simulink model "segway1"  (R2013a)
settings: Solver=ode45  StartTime=0.0  StopTime=10.0  RelTol=1e-3
values from neighbouring files (symbols this model uses):
  m = 0.05    [variables_set.m]
undefined symbols (not defined in the file or in its folder): Assem1, mass, platform, RootGround, RootPart, wheel
libraries: mblibv1 x13
settings Model: Creator=Raja  LastModifiedBy=Raja
settings SimMechanicsCC: VisOnUpdateDiagram=on  VisDuringSimulation=on

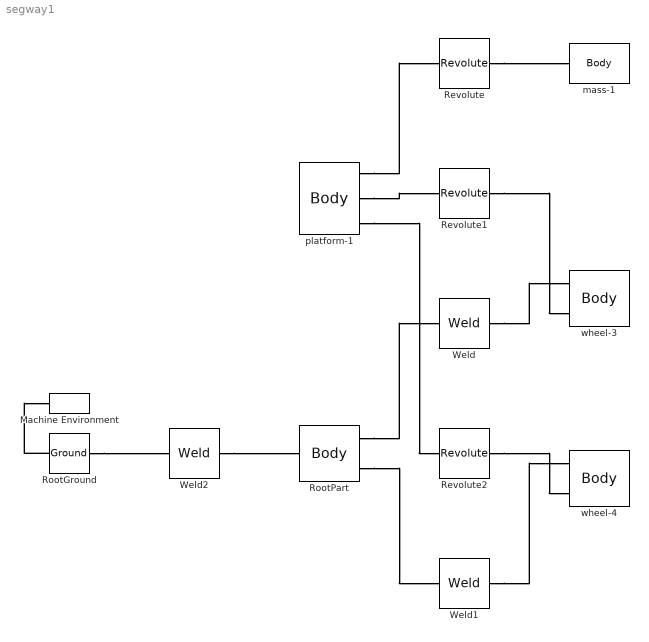
== system segway1 ==
  Machine Environment : mblibv1/Bodies/Machine Environment  PortType=env  PhysicalDomain=Mechanical  DialogTemplateClass=MECH.MachineEnvironment  SyncWhenCopied=off  Gravity=[0 -9.81 0]  GravityUnits=m/s^2  GravityAsSignal=off  Dimensionality=Auto-detect  AnalysisType=Forward dynamics  LinearAssemblyTolerance=1e-3  LinearAssemblyToleranceUnits=m  AngularAssemblyTolerance=1e-3  AngularAssemblyToleranceUnits=rad  ConstraintSolverType=Stabilizing  ConstraintRelTolerance=1e-4  ConstraintAbsTolerance=1e-4  UseRobustSingularityHandling=off  RedundancyAnalysisToleranceType=Automatically select tolerance  RedundancyAnalysisTolerance=1e-14  StatePerturbationType=Fixed  PerturbationSize=1e-5  VisualizeMachine=on  BodyVisualizationType=Use model default body geometries  BodyColorSelMode=Use model default  DefaultBodyColor=[1 0 0]
  Revolute : mblibv1/Joints/Revolute  LConnTagsString=__newl0  RConnTagsString=__newr0  UpdateFromCAD=on  PMImportedID=mass-1:-:platform-1  NumSAPorts=0  CutJoint=off  MarkAsCut=off  Primitives=prismatic  PrimitiveProps=R1$WORLD$[0,0.999884,-0.0152006]$revolute  DialogClass=JointBlock  R1Axis=[0,0.999884,-0.0152006]
  Revolute1 : mblibv1/Joints/Revolute  LConnTagsString=__newl0  RConnTagsString=__newr0  UpdateFromCAD=on  PMImportedID=platform-1:-:wheel-3  NumSAPorts=0  CutJoint=off  MarkAsCut=off  Primitives=prismatic  PrimitiveProps=R1$WORLD$[1,0,0]$revolute  DialogClass=JointBlock  R1Axis=[1,0,0]
  Revolute2 : mblibv1/Joints/Revolute  LConnTagsString=__newl0  RConnTagsString=__newr0  UpdateFromCAD=on  PMImportedID=platform-1:-:wheel-4  NumSAPorts=0  CutJoint=off  MarkAsCut=off  Primitives=prismatic  PrimitiveProps=R1$WORLD$[-1,0,0]$revolute  DialogClass=JointBlock  R1Axis=[-1,0,0]
  RootGround : mblibv1/Bodies/Ground  UpdateFromCAD=on  PMImportedID=RootGround  LeftPortType=env  RightPortType=workingframe  PhysicalDomain=Mechanical  DialogClass=GroundBlock  CoordPosition=[0,0.276214,-0.00378102]  CoordPositionUnits=m  StateVectorMgrId=-1  MachineId=[0 0]  ShowEnvPort=on
  RootPart : mblibv1/Bodies/Body  LConnTagsString=CS4  RConnTagsString=CS2|CS3  UpdateFromCAD=on  PMImportedID=Assem1/RootPart  DialogClass=MechanicalBodyBlock  Mass=0  MassUnits=kg  InertiaUnits=kg*m^2  Inertia=[0,0,0;0,0,0;0,0,0]  Shape=Cylinder  ShapeDims=[1 1]  ShapeUnits=m  ShapeUse=false  Density=1  DensityUnits=kg/m^3  DensityUse=false  GraphicsMode=MACHINE_DEFAULT  BodyColorSelMode=MACHINE_DEFAULT  BodyColor=[1;0;0]  AttachedToCS=CS1  CG=Right$CG$[0 0.276214 -0.00378102]$WORLD$WORLD$m$[1 0 0;0 1 0;0 0 1]$3x3 Transform$rad$WORLD$false$Assem1/RootPart::CG(AUTOGEN)  WorkingFrames=Right$CS1$[0 0 0]$WORLD$WORLD$m$[1 0 0;0 1 0;0 0 1]$3x3 Transform$rad$WORLD$false$Assem1/RootPart::CS1(AUTOGEN)#Right$CS2$[-0.15 0.0275 0]$WORLD$WORLD$m$[1 0 0;0 1 0;0 0 1]$3x3 Transform$rad$WORLD$true$Assem1/RootPart:-:wheel-3::Assem1/RootPart(AUTOGEN)#Right$CS3$[0.15 0.0275 0]$WORLD$WORLD$m$[1 0 0;0 1 0;0 0 1]$3x3 Transform$rad$WORLD$true$Assem1/RootPart:-:wheel-4::Assem1/RootPart(AUTOGEN)#Left$CS4$[0 0.276214 -0.00378102]$WORLD$WORLD$m$[1 0 0;0 1 0;0 0 1]$3x3 Transform$rad$WORLD$true$Assem1/RootPart:-:RootGround::Assem1/RootPart(AUTOGEN)  CGPos=[0 0.276214 -0.00378102]  CGRot=[1 0 0;0 1 0;0 0 1]  CS0Pos=[]  CS0Rot=[]  CS1Pos=[0 0 0]  CS1Rot=[1 0 0;0 1 0;0 0 1]  CS2Pos=[-0.15 0.0275 0]  CS2Rot=[1 0 0;0 1 0;0 0 1]  CS3Pos=[0.15 0.0275 0]  CS3Rot=[1 0 0;0 1 0;0 0 1]  CS4Pos=[0 0.276214 -0.00378102]  CS4Rot=[1 0 0;0 1 0;0 0 1]  CS5Pos=[]  CS5Rot=[]  CS6Pos=[]  CS6Rot=[]  CS7Pos=[]  CS7Rot=[]  CS8Pos=[]  CS8Rot=[]  CS9Pos=[]  CS9Rot=[]  CS10Pos=[]  CS10Rot=[]  CS11Pos=[]  CS11Rot=[]  CS12Pos=[]  CS12Rot=[]  CS13Pos=[]  CS13Rot=[]  CS14Pos=[]  CS14Rot=[]  CS15Pos=[]  CS15Rot=[]  CS16Pos=[]  CS16Rot=[]  CS17Pos=[]  CS17Rot=[]  CS18Pos=[]  CS18Rot=[]  CS19Pos=[]  CS19Rot=[]  CS20Pos=[]  CS20Rot=[]
  Weld : mblibv1/Joints/Weld  LConnTagsString=__newl0  RConnTagsString=__newr0  UpdateFromCAD=on  PMImportedID=Assem1/RootPart:-:wheel-3  NumSAPorts=0  CutJoint=off  MarkAsCut=off  Primitives=weld  PrimitiveProps=W$WORLD$[0.57735,0.57735,0.57735]$weld  DialogClass=JointBlock  WAxis=[0.57735,0.57735,0.57735]
  Weld1 : mblibv1/Joints/Weld  LConnTagsString=__newl0  RConnTagsString=__newr0  UpdateFromCAD=on  PMImportedID=Assem1/RootPart:-:wheel-4  NumSAPorts=0  CutJoint=off  MarkAsCut=off  Primitives=weld  PrimitiveProps=W$WORLD$[0.57735,0.57735,0.57735]$weld  DialogClass=JointBlock  WAxis=[0.57735,0.57735,0.57735]
  Weld2 : mblibv1/Joints/Weld  LConnTagsString=__newl0  RConnTagsString=__newr0  UpdateFromCAD=on  PMImportedID=Assem1/RootPart:-:RootGround  NumSAPorts=0  CutJoint=off  MarkAsCut=off  Primitives=weld  PrimitiveProps=W$WORLD$[0.57735,0.57735,0.57735]$weld  DialogClass=JointBlock  WAxis=[0.57735,0.57735,0.57735]
  mass-1 : mblibv1/Bodies/Body  LConnTagsString=CS2  UpdateFromCAD=on  PMImportedID=mass-1  DialogClass=MechanicalBodyBlock  Mass=0.994043  MassUnits=kg  InertiaUnits=kg*m^2  Inertia=[0.000433605,0,0;0,0.000718103,0;0,0,0.000433605]  Shape=Cylinder  ShapeDims=[1 1]  ShapeUnits=m  ShapeUse=false  Density=1  DensityUnits=kg/m^3  DensityUse=false  GraphicsMode=GFXFILE  GraphicsFileName=Assem1 - mass-1.STL  BodyColorSelMode=COLORPALETTE  BodyColor=[0.647059;0.619608;0.588235]  AttachedToCS=CS1  CG=Right$CG$[0 0.569937 -0.0082463]$WORLD$WORLD$m$[1 0 0;0 -0.999884 -0.0152006;0 0.0152006 -0.999884]$3x3 Transform$rad$WORLD$false$mass-1::CG(AUTOGEN)  WorkingFrames=Right$CS1$[0 0.584936 -0.00847431]$WORLD$WORLD$m$[1 0 0;0 -0.999884 -0.0152006;0 0.0152006 -0.999884]$3x3 Transform$rad$WORLD$false$mass-1::CS1(AUTOGEN)#Left$CS2$[0 0.554939 -0.00801829]$WORLD$WORLD$m$[1 0 0;0 1 0;0 0 1]$3x3 Transform$rad$WORLD$true$mass-1:-:platform-1::mass-1(AUTOGEN)  CGPos=[0 0.569937 -0.0082463]  CGRot=[1 0 0;0 -0.999884 -0.0152006;0 0.0152006 -0.999884]  CS0Pos=[]  CS0Rot=[]  CS1Pos=[0 0.584936 -0.00847431]  CS1Rot=[1 0 0;0 -0.999884 -0.0152006;0 0.0152006 -0.999884]  CS2Pos=[0 0.554939 -0.00801829]  CS2Rot=[1 0 0;0 1 0;0 0 1]  CS3Pos=[]  CS3Rot=[]  CS4Pos=[]  CS4Rot=[]  CS5Pos=[]  CS5Rot=[]  CS6Pos=[]  CS6Rot=[]  CS7Pos=[]  CS7Rot=[]  CS8Pos=[]  CS8Rot=[]  CS9Pos=[]  CS9Rot=[]  CS10Pos=[]  CS10Rot=[]  CS11Pos=[]  CS11Rot=[]  CS12Pos=[]  CS12Rot=[]  CS13Pos=[]  CS13Rot=[]  CS14Pos=[]  CS14Rot=[]  CS15Pos=[]  CS15Rot=[]  CS16Pos=[]  CS16Rot=[]  CS17Pos=[]  CS17Rot=[]  CS18Pos=[]  CS18Rot=[]  CS19Pos=[]  CS19Rot=[]  CS20Pos=[]  CS20Rot=[]
  platform-1 : mblibv1/Bodies/Body  RConnTagsString=CS2|CS3|CS4  UpdateFromCAD=on  PMImportedID=platform-1  DialogClass=MechanicalBodyBlock  Mass=0.91444  MassUnits=kg  InertiaUnits=kg*m^2  Inertia=[0.0247914,0,0;0,0.00462358,0;0,0,0.028624]  Shape=Cylinder  ShapeDims=[1 1]  ShapeUnits=m  ShapeUse=false  Density=1  DensityUnits=kg/m^3  DensityUse=false  GraphicsMode=GFXFILE  GraphicsFileName=Assem1 - platform-1.STL  BodyColorSelMode=COLORPALETTE  BodyColor=[0.866667;0.909804;1]  AttachedToCS=CS1  CG=Right$CG$[0 0.16518 -0.00209305]$WORLD$WORLD$m$[1 0 0;0 -0.999884 -0.0152006;0 0.0152006 -0.999884]$3x3 Transform$rad$WORLD$false$platform-1::CG(AUTOGEN)  WorkingFrames=Right$CS1$[0 0.0549968 -0.000418015]$WORLD$WORLD$m$[1 0 0;0 -0.999884 -0.0152006;0 0.0152006 -0.999884]$3x3 Transform$rad$WORLD$false$platform-1::CS1(AUTOGEN)#Right$CS2$[0 0.554939 -0.00801829]$WORLD$WORLD$m$[1 0 0;0 1 0;0 0 1]$3x3 Transform$rad$WORLD$true$mass-1:-:platform-1::platform-1(AUTOGEN)#Right$CS3$[-0.165 0.0275 0]$WORLD$WORLD$m$[1 0 0;0 1 0;0 0 1]$3x3 Transform$rad$WORLD$true$platform-1:-:wheel-3::platform-1(AUTOGEN)#Right$CS4$[0.165 0.0275 0]$WORLD$WORLD$m$[1 0 0;0 1 0;0 0 1]$3x3 Transform$rad$WORLD$true$platform-1:-:wheel-4::platform-1(AUTOGEN)  CGPos=[0 0.16518 -0.00209305]  CGRot=[1 0 0;0 -0.999884 -0.0152006;0 0.0152006 -0.999884]  CS0Pos=[]  CS0Rot=[]  CS1Pos=[0 0.0549968 -0.000418015]  CS1Rot=[1 0 0;0 -0.999884 -0.0152006;0 0.0152006 -0.999884]  CS2Pos=[0 0.554939 -0.00801829]  CS2Rot=[1 0 0;0 1 0;0 0 1]  CS3Pos=[-0.165 0.0275 0]  CS3Rot=[1 0 0;0 1 0;0 0 1]  CS4Pos=[0.165 0.0275 0]  CS4Rot=[1 0 0;0 1 0;0 0 1]  CS5Pos=[]  CS5Rot=[]  CS6Pos=[]  CS6Rot=[]  CS7Pos=[]  CS7Rot=[]  CS8Pos=[]  CS8Rot=[]  CS9Pos=[]  CS9Rot=[]  CS10Pos=[]  CS10Rot=[]  CS11Pos=[]  CS11Rot=[]  CS12Pos=[]  CS12Rot=[]  CS13Pos=[]  CS13Rot=[]  CS14Pos=[]  CS14Rot=[]  CS15Pos=[]  CS15Rot=[]  CS16Pos=[]  CS16Rot=[]  CS17Pos=[]  CS17Rot=[]  CS18Pos=[]  CS18Rot=[]  CS19Pos=[]  CS19Rot=[]  CS20Pos=[]  CS20Rot=[]
  wheel-3 : mblibv1/Bodies/Body  LConnTagsString=CS2|CS3  UpdateFromCAD=on  PMImportedID=wheel-3  DialogClass=MechanicalBodyBlock  Mass=0.38285  MassUnits=kg  InertiaUnits=kg*m^2  Inertia=[0.00079034,0,0;0,0.00042234,0;0,0,0.00042234]  Shape=Cylinder  ShapeDims=[1 1]  ShapeUnits=m  ShapeUse=false  Density=1  DensityUnits=kg/m^3  DensityUse=false  GraphicsMode=GFXFILE  GraphicsFileName=Assem1 - wheel-3.STL  BodyColorSelMode=COLORPALETTE  BodyColor=[0.294118;0.294118;0.294118]  AttachedToCS=CS1  CG=Right$CG$[-0.15 0.0275 0]$WORLD$WORLD$m$[1 0 0;0 1 0;0 0 1]$3x3 Transform$rad$WORLD$false$wheel-3::CG(AUTOGEN)  WorkingFrames=Right$CS1$[-0.165 0.0275 0]$WORLD$WORLD$m$[1 0 0;0 1 0;0 0 1]$3x3 Transform$rad$WORLD$false$wheel-3::CS1(AUTOGEN)#Left$CS2$[-0.15 0.0275 0]$WORLD$WORLD$m$[1 0 0;0 1 0;0 0 1]$3x3 Transform$rad$WORLD$true$Assem1/RootPart:-:wheel-3::wheel-3(AUTOGEN)#Left$CS3$[-0.165 0.0275 0]$WORLD$WORLD$m$[1 0 0;0 1 0;0 0 1]$3x3 Transform$rad$WORLD$true$platform-1:-:wheel-3::wheel-3(AUTOGEN)  CGPos=[-0.15 0.0275 0]  CGRot=[1 0 0;0 1 0;0 0 1]  CS0Pos=[]  CS0Rot=[]  CS1Pos=[-0.165 0.0275 0]  CS1Rot=[1 0 0;0 1 0;0 0 1]  CS2Pos=[-0.15 0.0275 0]  CS2Rot=[1 0 0;0 1 0;0 0 1]  CS3Pos=[-0.165 0.0275 0]  CS3Rot=[1 0 0;0 1 0;0 0 1]  CS4Pos=[]  CS4Rot=[]  CS5Pos=[]  CS5Rot=[]  CS6Pos=[]  CS6Rot=[]  CS7Pos=[]  CS7Rot=[]  CS8Pos=[]  CS8Rot=[]  CS9Pos=[]  CS9Rot=[]  CS10Pos=[]  CS10Rot=[]  CS11Pos=[]  CS11Rot=[]  CS12Pos=[]  CS12Rot=[]  CS13Pos=[]  CS13Rot=[]  CS14Pos=[]  CS14Rot=[]  CS15Pos=[]  CS15Rot=[]  CS16Pos=[]  CS16Rot=[]  CS17Pos=[]  CS17Rot=[]  CS18Pos=[]  CS18Rot=[]  CS19Pos=[]  CS19Rot=[]  CS20Pos=[]  CS20Rot=[]
  wheel-4 : mblibv1/Bodies/Body  LConnTagsString=CS2|CS3  UpdateFromCAD=on  PMImportedID=wheel-4  DialogClass=MechanicalBodyBlock  Mass=0.38285  MassUnits=kg  InertiaUnits=kg*m^2  Inertia=[0.00079034,0,0;0,0.00042234,0;0,0,0.00042234]  Shape=Cylinder  ShapeDims=[1 1]  ShapeUnits=m  ShapeUse=false  Density=1  DensityUnits=kg/m^3  DensityUse=false  GraphicsMode=GFXFILE  GraphicsFileName=Assem1 - wheel-4.STL  BodyColorSelMode=COLORPALETTE  BodyColor=[0.294118;0.294118;0.294118]  AttachedToCS=CS1  CG=Right$CG$[0.15 0.0275 0]$WORLD$WORLD$m$[1 0 0;0 1 0;0 0 1]$3x3 Transform$rad$WORLD$false$wheel-4::CG(AUTOGEN)  WorkingFrames=Right$CS1$[0.135 0.0275 0]$WORLD$WORLD$m$[1 0 0;0 1 0;0 0 1]$3x3 Transform$rad$WORLD$false$wheel-4::CS1(AUTOGEN)#Left$CS2$[0.15 0.0275 0]$WORLD$WORLD$m$[1 0 0;0 1 0;0 0 1]$3x3 Transform$rad$WORLD$true$Assem1/RootPart:-:wheel-4::wheel-4(AUTOGEN)#Left$CS3$[0.165 0.0275 0]$WORLD$WORLD$m$[1 0 0;0 1 0;0 0 1]$3x3 Transform$rad$WORLD$true$platform-1:-:wheel-4::wheel-4(AUTOGEN)  CGPos=[0.15 0.0275 0]  CGRot=[1 0 0;0 1 0;0 0 1]  CS0Pos=[]  CS0Rot=[]  CS1Pos=[0.135 0.0275 0]  CS1Rot=[1 0 0;0 1 0;0 0 1]  CS2Pos=[0.15 0.0275 0]  CS2Rot=[1 0 0;0 1 0;0 0 1]  CS3Pos=[0.165 0.0275 0]  CS3Rot=[1 0 0;0 1 0;0 0 1]  CS4Pos=[]  CS4Rot=[]  CS5Pos=[]  CS5Rot=[]  CS6Pos=[]  CS6Rot=[]  CS7Pos=[]  CS7Rot=[]  CS8Pos=[]  CS8Rot=[]  CS9Pos=[]  CS9Rot=[]  CS10Pos=[]  CS10Rot=[]  CS11Pos=[]  CS11Rot=[]  CS12Pos=[]  CS12Rot=[]  CS13Pos=[]  CS13Rot=[]  CS14Pos=[]  CS14Rot=[]  CS15Pos=[]  CS15Rot=[]  CS16Pos=[]  CS16Rot=[]  CS17Pos=[]  CS17Rot=[]  CS18Pos=[]  CS18Rot=[]  CS19Pos=[]  CS19Rot=[]  CS20Pos=[]  CS20Rot=[]
  connections:
  RootPart/RConn1 -- Weld/LConn1
  Weld/RConn1 -- wheel-3/LConn1
  RootPart/RConn2 -- Weld1/LConn1
  Weld1/RConn1 -- wheel-4/LConn1
  platform-1/RConn1 -- Revolute/LConn1
  Revolute/RConn1 -- mass-1/LConn1
  platform-1/RConn2 -- Revolute1/LConn1
  Revolute1/RConn1 -- wheel-3/LConn2
  platform-1/RConn3 -- Revolute2/LConn1
  Revolute2/RConn1 -- wheel-4/LConn2
  RootGround/RConn1 -- Weld2/LConn1
  Weld2/RConn1 -- RootPart/LConn1
  RootGround/LConn1 -- Machine Environment/RConn1
